simulink model "Final_Model_2025A"  (R2025a)
settings: Solver=VariableStepAuto  StartTime=0.0  StopTime=30  RelTol=1e-3
undefined symbols (not defined in the file): dspblkCoreblockFVToolHelper, gcbh
libraries: dsparch4 x6, dspvision x4, dspsnks4 x1
settings Model: Creator=harry  LastModifiedBy=hr563

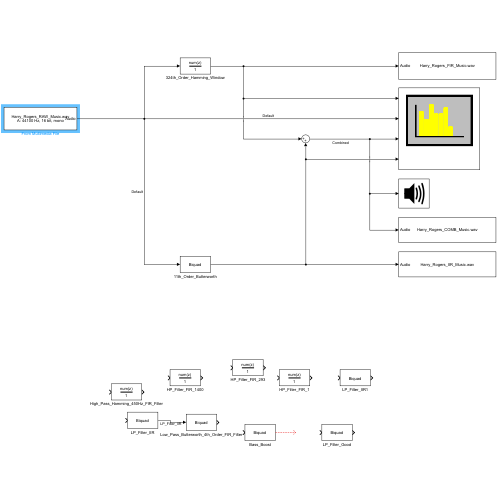
[thumbnail: Simulink's stored preview of the top-level diagram]
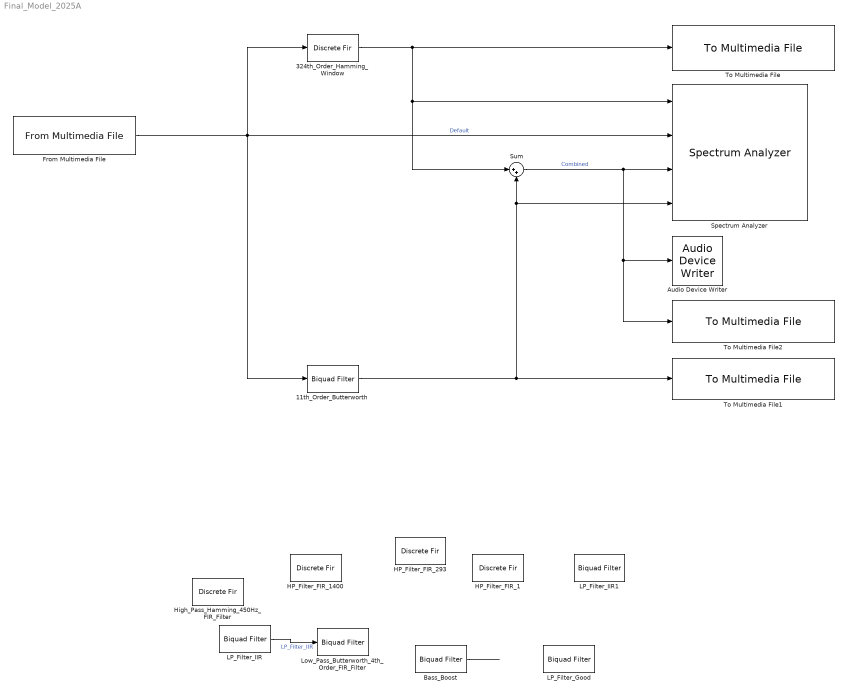
== system Final_Model_2025A ==
  11th_Order_Butterworth : dsparch4/Biquad Filter  Tag=BlockMethodSubSystem  FilterSource=Dialog parameters  CoeffSource=Specify via dialog  FilterObject=BQF  IIRFiltStruct=Direct form II  BiQuadCoeffs=[1 2 1 1 -1.86718651288637583 0.930317821620682883;1 2 1 1 -1.75017085842052844 0.809345759287786626;1 2 1 1 -1.65901358853543979 0.715106377514692082;1 2 1 1 -1.59437049097514039 0.648277636837619742;1 2 1 1 -1.55591215178388231 0.60851898550928496;1 1 0 1 -0.771580047210876474 0]  ScaleValues=[0.0157828271835766983;0.0147937252168145895;0.0140231972448130234;0.0134767864656198163;0.0131517084313506494;0.114209976394561735;1]  IC=0  ICnum=0  ICden=0  a0Flag=Warning  optimizeScaleValues=on  ScaleValueMode=Specify via input port (g)  InputProcessing=Columns as channels (frame based)  roundingMode=Floor  overflowMode=off  scaleValueFracLength=14  denProdOutputFracLength=30  denAccumFracLength=30  secondMemoryFracLength=15
  324th_Order_Hamming_Window : DiscreteFir  Tag=BlockMethodSubSystem  Coefficients=[0.000101883144796532701 6.86919896372373761e-05 3.0551827126106626e-05 -1.03598348954163603e-05 -5.16579270239632391e-05 -9.08628616463472204e-05 -0.000125523401849254363 -0.000153345544928162425 -0.000172322705682308142 -0.0001808615327952031 -0.000177896814554488319 -0.000162988272937909177 -0.000136391758987141042 -9.90975869556805417e-05 -5.28295892007051579e-05 3.67373583371040851e-19 5.63825150002342541e-05 0.000112851545613355976 0.000165664909834257676 0.000211022928791822369 0.000245312472036879933 0.000265363001797536201 0.000268698231497241239 0.000253765330008578279 0.000220123109025119166 0.000168571515594089758 0.000101207108725427596 2.13930078590154471e-05 -6.63630819330360814e-05 -0.000156623005104577644 -0.000243317869524272844 -0.000320119750054912008 -0.000380865129789689934 -0.000420004064119163347 -0.000433044725249857616 -0.000416960561512023258 -0.000370527146366229139 -0.000294558108627706922 -0.00019201436393307482 -6.79680504334934652e-05 7.05882443586693624e-05 0.000215085730591075002 0.000355864481977990078 0.000482775278779599786 0.000585863696247650189 0.000656093174251949737 0.000686057617941617914 0.000670631094018952763 0.000607502860797922524 0.000497550517162741808 0.000345012413622010296 0.000157432285192392427 -5.46362948927894444e-05 -0.000278161469031175032 -0.000498379071641175272 -0.000699714415808812555 -0.000866825914804108871 -0.00098570410124290621 -0.00104475114779683078 -0.0010357624136966496 -0.000954733413222053073 -0.000802423133919360218 -0.000584617630106775408 -0.000312055677203152706 -3.65606249683564421e-17 0.000332538151684784098 0.000663888110730826049 0.000971065241568101474 0.00123129363830265254 0.00142360956883102498 0.00153043758852049573 0.00153902667756687303 0.00144263691875525283 0.00124137834252432836 0.000942622283484140732 0.000560931015285178478 0.000117482131024904072 -0.000361001765768432072 -0.000843772220868447783 -0.00129794307480813687 -0.0016906374133820437 -0.00199125886818211266 -0.00217373660619727196 -0.00221858677488572832 -0.00211463719958366768 -0.00186027704044082454 -0.00146411843666072942 -0.00094499167688704398 -0.000331237214998534777 0.000340695622130973491 0.00102828509125300438 0.00168550368985615059 0.00226576801035194113 0.00272509066434238655 0.0030252296844812134 0.00313662014587347141 0.00304087624971733066 0.00273267024058921172 0.00222082676923184442 0.0015285161619500217 0.000692485083967047787 -0.000238674949218946607 -0.00120715570869207411 -0.00214932764463113832 -0.00299971477484106555 -0.00369531265232305546 -0.00417997777328447256 -0.00440859799464370788 -0.00435075319633216034 -0.00399359443685079994 -0.00334370785079183197 -0.00242778488815178616 -0.0012919903404852379 9.92606710287512014e-17 0.00137023404897434337 0.0027308459883259948 0.00398932091309959873 0.00505436537057680092 0.00584203302811834874 0.00628172024669043216 0.00632163509487150988 0.00593335705089946108 0.00511514350829275332 0.00389370181746993838 0.00232422898026746075 0.000488620844677755198 -0.00150813690696118105 -0.00354326904389297512 -0.00548296361206709534 -0.0071902367066978487 -0.00853348343040164631 -0.00939522672770957447 -0.00968054059413358745 -0.00932461951342663208 -0.0082989932880848296 -0.0066159451763069272 -0.00433077896314346209 -0.00154169294984985664 0.00161285011947875641 0.00495922573952324586 0.00829604582443028982 0.0114035350094972912 0.0140544413260888078 0.016025932931825377 0.0171118565994586753 0.0171346915278984546 0.0159565270886542591 0.0134884265742894315 0.00969760983343864909 0.00461199258818189954 -0.00167824611344687927 -0.00902224159297380576 -0.0172131713291425285 -0.0259959658054706444 -0.0350776695661746893 -0.0441399695405789508 -0.0528532821217139182 -0.0608916968874572279 -0.0679480189210882463 -0.0737481369847406143 -0.0780639725324154959 -0.0807243334855240052 0.918259911176981802 -0.0807243334855240052 -0.0780639725324154959 -0.0737481369847406143 -0.0679480189210882463 -0.0608916968874572279 ...(+3741 chars)]  InputProcessing=Columns as channels (frame based)
  Audio Device Writer : dspsnks4/Audio Device Writer  Driver=DirectSound  Device=Default  InheritSampleRate=on  SampleRate=44100  BitDepth=16-bit integer  BufferSize=4096  NumBuffers=10  DefaultOutputChannelMapping=on  OutputChannelMapping=1:2  OutputNumUnderrunSamples=off  DriverIdx=1  DeviceWarnFlag=''
  Bass_Boost : dsparch4/Biquad Filter  Tag=BlockMethodSubSystem  FilterSource=Dialog parameters  CoeffSource=Specify via dialog  FilterObject=BQF  IIRFiltStruct=Direct form II  BiQuadCoeffs=[1 0 -1 1 -1.97922777247152193 0.979852553935027126;1 0 -1 1 -1.99208152287231277 0.992175167997945806]  ScaleValues=[0.0099035520411623959;0.0099035520411623959;1]  IC=0  ICnum=0  ICden=0  a0Flag=Warning  optimizeScaleValues=on  ScaleValueMode=Specify via input port (g)  InputProcessing=Columns as channels (frame based)  roundingMode=Floor  overflowMode=off  scaleValueFracLength=14  denProdOutputFracLength=30  denAccumFracLength=30  secondMemoryFracLength=15
  From Multimedia File : dspvision/From Multimedia File  inputFilename=C:\Users\hr563\OneDrive - University of Brighton\Year 3\EO626 - Digital Signal Processing\02 - Labs & Coursework\Final Project\Version 2\Harry_Rogers_RAW_Music.wav  readRange=[1 Inf]  loop=on  numPlays=inf  outputStreams=Audio only  videoDataType=single  audioDataType=double  inheritSampleTime=on  userDefinedSampleTime=1/30  noAudioOutput=off  isIntensityVideo=off  fourcc=RGB  colorVideoFormat=Separate color signals  outputEOF=off  dataOrg=Column-major  audioFrameSize=1024  computeAudioFrameSize=off  outSamplingMode=Sample based
      settings: LibrarySourceBlock=audiosources/From Multimedia File
  HP_Filter_FIR_1 : DiscreteFir  Tag=BlockMethodSubSystem  LoadFcn=dspblkCoreblockFVToolHelper(gcbh,'load');  Coefficients=[-0.000172363924315728858 -0.000162411128573225228 -0.000141952632408346325 -0.000111937875448206057 -7.3851199371037808e-05 -2.9665348286780504e-05 1.82276088386097535e-05 6.71088533093024717e-05 0.000114048947032513665 0.000156046191835491031 0.000190184041238055756 0.000213802202744505318 0.000224673747451289524 0.000221178337738877408 0.000202459872990196294 0.000168555718425642166 0.00012048447429225332 6.028015285343048e-05 -9.0372368165297075e-06 -8.35613444034827242e-05 -0.000158671573688910707 -0.00022927451432170617 -0.000290105803670732206 -0.00033607765210802253 -0.000362651848377851607 -0.000366213607692528946 -0.000344418626364605509 -0.000296484582778010057 -0.000223399378251365769 -0.000128021791785200718 -1.50558976478667982e-05 0.000109111662719308189 0.000236713072915811486 0.000359030473486977799 0.000466937148628223774 0.000551518831532300346 0.00060473630847924717 0.000620083808060237435 0.000593193875587250813 0.000522339099862775304 0.000408784497940755179 0.000256951620138050395 7.43662639955295377e-05 -0.000128624463839541327 -0.000339363947310907747 -0.000543607733929659981 -0.000726418970532887506 -0.000873185750649687546 -0.00097069545809302135 -0.00100819198737314882 -0.000978337351840312657 -0.000878000331284546111 -0.000708801768935293699 -0.000477358793517133125 -0.000195188069684670715 0.000121749798270892953 0.000453857713884555042 0.000779028316384048161 0.00107403047870383993 0.00131607467262399532 0.00148445729625005574 0.00156217158522543474 0.00153736757952660334 0.00140454663245319919 0.00116538742266552317 0.000829120060655970186 0.000412391753901741398 -6.1399883169818039e-05 -0.000563293414391254467 -0.00106041986086509075 -0.00151804198472996221 -0.00190185733672405539 -0.00218041976363849256 -0.00232751673198150662 -0.0023243329454521555 -0.00216123540699293031 -0.00183903163276229165 -0.00136958067386139899 -0.000775674619164995385 -9.01542351587077237e-05 0.000645726430807490163 0.00138461858811187648 0.00207596111382843222 0.0026692615626617653 0.00311757334470875091 0.00338094138492120054 0.00342957760910434211 0.00324653243692826689 0.0028296496090265558 0.00219262854278050659 0.00136506930185104698 0.000391437435900149648 -0.000671044248027770178 -0.00175549682802994393 -0.00278932756878535072 -0.00369879642900174674 -0.00441393573992427627 -0.00487351324290121596 -0.00502970856114155936 -0.00485217399934524153 -0.00433117329036738705 -0.0034795361035329553 -0.00233322991392799408 -0.000950430945598244176 0.00059093213758860052 0.00219708976874827787 0.00376362758981319207 0.0051817039743920143 0.00634494566982728332 0.00715661624830996653 0.00753661293967718832 0.00742783471297681595 0.00680148013467851177 0.00566087777367077494 0.00404352314560369255 0.00202109101148037224 -0.000302694738201085491 -0.00279632574162053766 -0.00530677000518562855 -0.00766746317937382679 -0.00970764829638974015 -0.0112625845722653661 -0.012184074032272273 -0.0123507139156610306 -0.0116772768537853379 -0.0101226515937356768 -0.00769584445638855572 -0.00445964373969970612 -0.00053168220654616744 0.00391720821819646972 0.00866727552988320188 0.0134564898180329438 0.0179890652298531316 0.0219451435763498778 0.0249906435928888039 0.0267859088499742271 0.0269912108286908779 0.0252661306287800883 0.0212577699554858598 0.0145681863422995467 0.00468052310781379068 -0.00920564171979430454 -0.0285662975876889227 -0.0566203819789594456 -0.101953907686601439 -0.196616698385724042 -0.631266180659922238 0.631266180659922238 0.196616698385724042 0.101953907686601439 0.0566203819789594456 0.0285662975876889227 0.00920564171979430454 -0.00468052310781379068 -0.0145681863422995467 -0.0212577699554858598 -0.0252661306287800883 -0.0269912108286908779 -0.0267859088499742271 -0.0249906435928888039 -0.0219451435763498778 -0.0179890652298531316 -0.0134564898180329438 -0.00866727552988320188 -0.00391720821819646972 0.00053168220654616744 0.00445964373969970612 0.00769584445638855572 0.0101226515937356768 ...(+2982 chars)]  InputProcessing=Columns as channels (frame based)
      settings: CopyFcn=dspblkCoreblockFVToolHelper(gcbh,'copy');  DeleteFcn=dspblkCoreblockFVToolHelper(gcbh,'close');  ModelCloseFcn=dspblkCoreblockFVToolHelper(gcbh,'close');  PreSaveFcn=dspblkCoreblockFVToolHelper(gcbh,'presave');  PostSaveFcn=dspblkCoreblockFVToolHelper(gcbh,'postsave');  CloseFcn=dspblkCoreblockFVToolHelper(gcbh,'close');
  HP_Filter_FIR_1400 : DiscreteFir  Tag=BlockMethodSubSystem  Coefficients=[-3.41011682905011137e-05 -3.10559172244132767e-05 -2.59704425703152653e-05 -1.91699897519594766e-05 -1.10922885580064924e-05 -2.25957592028960039e-06 6.75493320791177441e-06 1.5363989756872894e-05 2.30043051885164215e-05 2.91731560537851625e-05 3.34612364628995916e-05 3.55796265981361698e-05 3.53791128579665512e-05 3.28605772797087772e-05 2.817574042505612e-05 2.16181572859737575e-05 1.36049910339950962e-05 4.65068479285764637e-06 -4.6658210837113406e-06 -1.37382535674786507e-05 -2.19721854293832492e-05 -2.88237141255762545e-05 -3.38351420219722165e-05 -3.66653335945134315e-05 -3.71127502897256254e-05 -3.51296195208254772e-05 -3.08262527275190195e-05 -2.44651536838152741e-05 -1.64452128142218818e-05 -7.27692453362485335e-06 2.44984861227346711e-06 1.21035470412975323e-05 2.10516334209167097e-05 2.87017539985367584e-05 3.45406822275087029e-05 3.81685019521315502e-05 3.93257692886763203e-05 3.79118227132474732e-05 3.39929636933614958e-05 2.77998712973231524e-05 1.97143033587088446e-05 1.02458301928054272e-05 -1.43291443473674532e-18 -1.03600945567594416e-05 -2.01564292519422879e-05 -2.87401223854129503e-05 -3.55341248592242601e-05 -4.00717364834981459e-05 -4.20283952608714961e-05 -4.12445910286335254e-05 -3.77383036428625458e-05 -3.17060253166553859e-05 -2.35121556387111352e-05 -1.36673100192635751e-05 -2.79680951490947161e-06 8.39872521177538563e-06 1.91882140173775877e-05 2.88575429812699572e-05 3.67565199570511276e-05 4.23422925095269241e-05 4.5216348115168936e-05 4.51525936634749101e-05 4.21145565924994767e-05 3.62604305214517085e-05 2.79354618385117793e-05 1.76519915136439117e-05 6.05827596191914808e-06 -6.10204067022114899e-06 -1.80372925035369491e-05 -2.89590018398164513e-05 -3.81336422904404674e-05 -4.49315780750668805e-05 -4.88699350290324068e-05 -4.96465052091935567e-05 -4.71623279491193041e-05 -4.15312936419230796e-05 -3.30759391668579956e-05 -2.23094939846204235e-05 -9.90513650925184875e-06 3.345727209407499e-06 1.65836026605182578e-05 2.89363114943004043e-05 3.95761131366971562e-05 4.77748246071605157e-05 5.2953290051345063e-05 5.47218618906218475e-05 5.29090897148440042e-05 4.75765399293508288e-05 3.90185443937111727e-05 2.77466450637399063e-05 1.44595020988057325e-05 -1.18271311595691961e-18 -1.4697843873563345e-05 -2.86688503206844876e-05 -4.09797025741088575e-05 -5.07909318547471202e-05 -5.74137706463406609e-05 -6.03580474054663733e-05 -5.93678196977923654e-05 -5.44421921531140565e-05 -4.58396959021705236e-05 -3.40656593559356003e-05 -1.98431092620320828e-05 -4.0688340026943614e-06 1.22427540683630008e-05 2.80244714637696102e-05 4.22258112556728377e-05 5.38824907874365126e-05 6.21815193377174091e-05 6.65174204924286102e-05 6.65357500618489879e-05 6.21608195978629133e-05 5.36055219630269039e-05 4.13622978888251875e-05 2.61755085599021872e-05 8.99670967999697371e-06 -9.07452379900674041e-06 -2.68605734952090588e-05 -4.31821283474038999e-05 -5.69359858632199542e-05 -6.71691965022533729e-05 -7.31445945383622976e-05 -7.43932391404152651e-05 -7.07500737262434655e-05 -6.23701535911282064e-05 -4.97240272600675692e-05 -3.3572207898318735e-05 -1.49200503392781792e-05 5.04433369426768165e-06 2.50253228685259366e-05 4.37034600126417734e-05 5.98221757188546798e-05 7.22718881018664206e-05 8.01658775142756556e-05 8.29027787878004025e-05 8.02113259973277195e-05 7.21740797205544483e-05 5.92281973553958766e-05 4.21427895438527663e-05 2.19739448675932221e-05 -2.99731528384923268e-18 -2.23590162023749559e-05 -4.36327205209957573e-05 -6.23966489100494638e-05 -7.73671897462060315e-05 -8.74888783155105995e-05 -9.20081476517277489e-05 -9.05284218871913311e-05 -8.30425815327852059e-05 -6.99402562086595512e-05 -5.19890199878336265e-05 -3.02902739761851766e-05 -6.21228852709459262e-06 1.86955684798287861e-05 4.28020757771411278e-05 6.45005488484745853e-05 8.2315465957998396e-05 9.50022831821261413e-05 0.000101633718625495422 0.000101666563444777433 9.49842615824907457e-05 8.19120199887399361e-05 6.32029718649274248e-05 ...(+31187 chars)]  InputProcessing=Columns as channels (frame based)
  HP_Filter_FIR_293 : DiscreteFir  Tag=BlockMethodSubSystem  LoadFcn=dspblkCoreblockFVToolHelper(gcbh,'load');  Coefficients=[-0.000172363924315728858 -0.000162411128573225228 -0.000141952632408346325 -0.000111937875448206057 -7.3851199371037808e-05 -2.9665348286780504e-05 1.82276088386097535e-05 6.71088533093024717e-05 0.000114048947032513665 0.000156046191835491031 0.000190184041238055756 0.000213802202744505318 0.000224673747451289524 0.000221178337738877408 0.000202459872990196294 0.000168555718425642166 0.00012048447429225332 6.028015285343048e-05 -9.0372368165297075e-06 -8.35613444034827242e-05 -0.000158671573688910707 -0.00022927451432170617 -0.000290105803670732206 -0.00033607765210802253 -0.000362651848377851607 -0.000366213607692528946 -0.000344418626364605509 -0.000296484582778010057 -0.000223399378251365769 -0.000128021791785200718 -1.50558976478667982e-05 0.000109111662719308189 0.000236713072915811486 0.000359030473486977799 0.000466937148628223774 0.000551518831532300346 0.00060473630847924717 0.000620083808060237435 0.000593193875587250813 0.000522339099862775304 0.000408784497940755179 0.000256951620138050395 7.43662639955295377e-05 -0.000128624463839541327 -0.000339363947310907747 -0.000543607733929659981 -0.000726418970532887506 -0.000873185750649687546 -0.00097069545809302135 -0.00100819198737314882 -0.000978337351840312657 -0.000878000331284546111 -0.000708801768935293699 -0.000477358793517133125 -0.000195188069684670715 0.000121749798270892953 0.000453857713884555042 0.000779028316384048161 0.00107403047870383993 0.00131607467262399532 0.00148445729625005574 0.00156217158522543474 0.00153736757952660334 0.00140454663245319919 0.00116538742266552317 0.000829120060655970186 0.000412391753901741398 -6.1399883169818039e-05 -0.000563293414391254467 -0.00106041986086509075 -0.00151804198472996221 -0.00190185733672405539 -0.00218041976363849256 -0.00232751673198150662 -0.0023243329454521555 -0.00216123540699293031 -0.00183903163276229165 -0.00136958067386139899 -0.000775674619164995385 -9.01542351587077237e-05 0.000645726430807490163 0.00138461858811187648 0.00207596111382843222 0.0026692615626617653 0.00311757334470875091 0.00338094138492120054 0.00342957760910434211 0.00324653243692826689 0.0028296496090265558 0.00219262854278050659 0.00136506930185104698 0.000391437435900149648 -0.000671044248027770178 -0.00175549682802994393 -0.00278932756878535072 -0.00369879642900174674 -0.00441393573992427627 -0.00487351324290121596 -0.00502970856114155936 -0.00485217399934524153 -0.00433117329036738705 -0.0034795361035329553 -0.00233322991392799408 -0.000950430945598244176 0.00059093213758860052 0.00219708976874827787 0.00376362758981319207 0.0051817039743920143 0.00634494566982728332 0.00715661624830996653 0.00753661293967718832 0.00742783471297681595 0.00680148013467851177 0.00566087777367077494 0.00404352314560369255 0.00202109101148037224 -0.000302694738201085491 -0.00279632574162053766 -0.00530677000518562855 -0.00766746317937382679 -0.00970764829638974015 -0.0112625845722653661 -0.012184074032272273 -0.0123507139156610306 -0.0116772768537853379 -0.0101226515937356768 -0.00769584445638855572 -0.00445964373969970612 -0.00053168220654616744 0.00391720821819646972 0.00866727552988320188 0.0134564898180329438 0.0179890652298531316 0.0219451435763498778 0.0249906435928888039 0.0267859088499742271 0.0269912108286908779 0.0252661306287800883 0.0212577699554858598 0.0145681863422995467 0.00468052310781379068 -0.00920564171979430454 -0.0285662975876889227 -0.0566203819789594456 -0.101953907686601439 -0.196616698385724042 -0.631266180659922238 0.631266180659922238 0.196616698385724042 0.101953907686601439 0.0566203819789594456 0.0285662975876889227 0.00920564171979430454 -0.00468052310781379068 -0.0145681863422995467 -0.0212577699554858598 -0.0252661306287800883 -0.0269912108286908779 -0.0267859088499742271 -0.0249906435928888039 -0.0219451435763498778 -0.0179890652298531316 -0.0134564898180329438 -0.00866727552988320188 -0.00391720821819646972 0.00053168220654616744 0.00445964373969970612 0.00769584445638855572 0.0101226515937356768 ...(+2982 chars)]  InputProcessing=Columns as channels (frame based)
      settings: CopyFcn=dspblkCoreblockFVToolHelper(gcbh,'copy');  DeleteFcn=dspblkCoreblockFVToolHelper(gcbh,'close');  ModelCloseFcn=dspblkCoreblockFVToolHelper(gcbh,'close');  PreSaveFcn=dspblkCoreblockFVToolHelper(gcbh,'presave');  PostSaveFcn=dspblkCoreblockFVToolHelper(gcbh,'postsave');  CloseFcn=dspblkCoreblockFVToolHelper(gcbh,'close');
  High_Pass_Hamming_450Hz_FIR_Filter : DiscreteFir  Tag=BlockMethodSubSystem  Coefficients=[0.000101883144796532701 6.86919896372373761e-05 3.0551827126106626e-05 -1.03598348954163603e-05 -5.16579270239632391e-05 -9.08628616463472204e-05 -0.000125523401849254363 -0.000153345544928162425 -0.000172322705682308142 -0.0001808615327952031 -0.000177896814554488319 -0.000162988272937909177 -0.000136391758987141042 -9.90975869556805417e-05 -5.28295892007051579e-05 3.67373583371040851e-19 5.63825150002342541e-05 0.000112851545613355976 0.000165664909834257676 0.000211022928791822369 0.000245312472036879933 0.000265363001797536201 0.000268698231497241239 0.000253765330008578279 0.000220123109025119166 0.000168571515594089758 0.000101207108725427596 2.13930078590154471e-05 -6.63630819330360814e-05 -0.000156623005104577644 -0.000243317869524272844 -0.000320119750054912008 -0.000380865129789689934 -0.000420004064119163347 -0.000433044725249857616 -0.000416960561512023258 -0.000370527146366229139 -0.000294558108627706922 -0.00019201436393307482 -6.79680504334934652e-05 7.05882443586693624e-05 0.000215085730591075002 0.000355864481977990078 0.000482775278779599786 0.000585863696247650189 0.000656093174251949737 0.000686057617941617914 0.000670631094018952763 0.000607502860797922524 0.000497550517162741808 0.000345012413622010296 0.000157432285192392427 -5.46362948927894444e-05 -0.000278161469031175032 -0.000498379071641175272 -0.000699714415808812555 -0.000866825914804108871 -0.00098570410124290621 -0.00104475114779683078 -0.0010357624136966496 -0.000954733413222053073 -0.000802423133919360218 -0.000584617630106775408 -0.000312055677203152706 -3.65606249683564421e-17 0.000332538151684784098 0.000663888110730826049 0.000971065241568101474 0.00123129363830265254 0.00142360956883102498 0.00153043758852049573 0.00153902667756687303 0.00144263691875525283 0.00124137834252432836 0.000942622283484140732 0.000560931015285178478 0.000117482131024904072 -0.000361001765768432072 -0.000843772220868447783 -0.00129794307480813687 -0.0016906374133820437 -0.00199125886818211266 -0.00217373660619727196 -0.00221858677488572832 -0.00211463719958366768 -0.00186027704044082454 -0.00146411843666072942 -0.00094499167688704398 -0.000331237214998534777 0.000340695622130973491 0.00102828509125300438 0.00168550368985615059 0.00226576801035194113 0.00272509066434238655 0.0030252296844812134 0.00313662014587347141 0.00304087624971733066 0.00273267024058921172 0.00222082676923184442 0.0015285161619500217 0.000692485083967047787 -0.000238674949218946607 -0.00120715570869207411 -0.00214932764463113832 -0.00299971477484106555 -0.00369531265232305546 -0.00417997777328447256 -0.00440859799464370788 -0.00435075319633216034 -0.00399359443685079994 -0.00334370785079183197 -0.00242778488815178616 -0.0012919903404852379 9.92606710287512014e-17 0.00137023404897434337 0.0027308459883259948 0.00398932091309959873 0.00505436537057680092 0.00584203302811834874 0.00628172024669043216 0.00632163509487150988 0.00593335705089946108 0.00511514350829275332 0.00389370181746993838 0.00232422898026746075 0.000488620844677755198 -0.00150813690696118105 -0.00354326904389297512 -0.00548296361206709534 -0.0071902367066978487 -0.00853348343040164631 -0.00939522672770957447 -0.00968054059413358745 -0.00932461951342663208 -0.0082989932880848296 -0.0066159451763069272 -0.00433077896314346209 -0.00154169294984985664 0.00161285011947875641 0.00495922573952324586 0.00829604582443028982 0.0114035350094972912 0.0140544413260888078 0.016025932931825377 0.0171118565994586753 0.0171346915278984546 0.0159565270886542591 0.0134884265742894315 0.00969760983343864909 0.00461199258818189954 -0.00167824611344687927 -0.00902224159297380576 -0.0172131713291425285 -0.0259959658054706444 -0.0350776695661746893 -0.0441399695405789508 -0.0528532821217139182 -0.0608916968874572279 -0.0679480189210882463 -0.0737481369847406143 -0.0780639725324154959 -0.0807243334855240052 0.918259911176981802 -0.0807243334855240052 -0.0780639725324154959 -0.0737481369847406143 -0.0679480189210882463 -0.0608916968874572279 ...(+3741 chars)]  InputProcessing=Columns as channels (frame based)
  LP_Filter_Good : dsparch4/Biquad Filter  Tag=BlockMethodSubSystem  FilterSource=Dialog parameters  CoeffSource=Specify via dialog  FilterObject=BQF  IIRFiltStruct=Direct form II  BiQuadCoeffs=[1 2 1 1 -1.76341598268706057 0.823038713497136087;1 2 1 1 -1.56729903101675361 0.620290865695949267]  ScaleValues=[0.0149056827025188555;0.0132479586697988976;1]  IC=0  ICnum=0  ICden=0  a0Flag=Warning  optimizeScaleValues=on  ScaleValueMode=Specify via input port (g)  InputProcessing=Columns as channels (frame based)  roundingMode=Floor  overflowMode=off  scaleValueFracLength=14  denProdOutputFracLength=30  denAccumFracLength=30  secondMemoryFracLength=15
  LP_Filter_IIR : dsparch4/Biquad Filter  Tag=BlockMethodSubSystem  FilterSource=Dialog parameters  CoeffSource=Specify via dialog  FilterObject=BQF  IIRFiltStruct=Direct form II  BiQuadCoeffs=[1 2 1 1 -1.83393339064791361 0.886044963112266548;1 2 1 1 -1.6692031429311931 0.716633873504157637;1 2 1 1 -1.5869067908315011 0.631999054621612988]  ScaleValues=[0.0130278931160882541;0.0118576826432411561;0.011273065947527923;1]  IC=0  ICnum=0  ICden=0  a0Flag=Warning  optimizeScaleValues=on  ScaleValueMode=Specify via input port (g)  InputProcessing=Columns as channels (frame based)  roundingMode=Floor  overflowMode=off  scaleValueFracLength=14  denProdOutputFracLength=30  denAccumFracLength=30  secondMemoryFracLength=15
  LP_Filter_IIR1 : dsparch4/Biquad Filter  Tag=BlockMethodSubSystem  FilterSource=Dialog parameters  CoeffSource=Specify via dialog  FilterObject=BQF  IIRFiltStruct=Direct form II  BiQuadCoeffs=[1 2 1 1 -1.83393339064791361 0.886044963112266548;1 2 1 1 -1.6692031429311931 0.716633873504157637;1 2 1 1 -1.5869067908315011 0.631999054621612988]  ScaleValues=[0.0130278931160882541;0.0118576826432411561;0.011273065947527923;1]  IC=0  ICnum=0  ICden=0  a0Flag=Warning  optimizeScaleValues=on  ScaleValueMode=Specify via input port (g)  InputProcessing=Columns as channels (frame based)  roundingMode=Floor  overflowMode=off  scaleValueFracLength=14  denProdOutputFracLength=30  denAccumFracLength=30  secondMemoryFracLength=15
  Low_Pass_Butterworth_4th_Order_FIR_Filter : dsparch4/Biquad Filter  Tag=BlockMethodSubSystem  FilterSource=Dialog parameters  CoeffSource=Specify via dialog  FilterObject=BQF  IIRFiltStruct=Direct form II  BiQuadCoeffs=[1 2 1 1 -1.76341598268706057 0.823038713497136087;1 2 1 1 -1.56729903101675361 0.620290865695949267]  ScaleValues=[0.0149056827025188555;0.0132479586697988976;1]  IC=0  ICnum=0  ICden=0  a0Flag=Warning  optimizeScaleValues=on  ScaleValueMode=Specify via input port (g)  InputProcessing=Columns as channels (frame based)  roundingMode=Floor  overflowMode=off  scaleValueFracLength=14  denProdOutputFracLength=30  denAccumFracLength=30  secondMemoryFracLength=15
  Spectrum Analyzer : SpectrumAnalyzer  NumInputPorts=4  WindowPosition=[130.000000,32.000000,1675.000000,849.000000,]  ScopeFrameLocation=window  SampleRate=44.1e3  FrequencyScale=Log  WindowInvariantSamplesPerUpdate=on  FrequencySpan=Start and stop frequencies  StartFrequency=20  StopFrequency=22050  MaximizeAxes=Off  YLimits=[-277.2722 31.5803]  ShowLegend=on  ExpandToolstrip=on  SelectedToolstripTab=spectrumAnalyzerToolstrip.channelMeasurementsTab  MeasurementChannel=0
  Sum : Sum  Inputs=|++
  To Multimedia File : dspvision/To Multimedia File  outputFilename=Harry_Rogers_FIR_Music.wav  streamSelection=Audio only  videoCompressor=None (uncompressed)  audioCompressor=None (uncompressed)  imagePorts=One multidimensional signal  fileType=WAV  audioDatatype=16-bit integer  fourcc=RGB  audioBitRate=128  audioQuality=75  videoQuality=75  mj2000CompFactor=10
      settings: LibrarySourceBlock=audiosinks/To Multimedia File
  To Multimedia File1 : dspvision/To Multimedia File  outputFilename=Harry_Rogers_IIR_Music.wav  streamSelection=Audio only  videoCompressor=None (uncompressed)  audioCompressor=None (uncompressed)  imagePorts=One multidimensional signal  fileType=WAV  audioDatatype=16-bit integer  fourcc=RGB  audioBitRate=128  audioQuality=75  videoQuality=75  mj2000CompFactor=10
      settings: LibrarySourceBlock=audiosinks/To Multimedia File
  To Multimedia File2 : dspvision/To Multimedia File  outputFilename=Harry_Rogers_COMB_Music.wav  streamSelection=Audio only  videoCompressor=None (uncompressed)  audioCompressor=None (uncompressed)  imagePorts=One multidimensional signal  fileType=WAV  audioDatatype=16-bit integer  fourcc=RGB  audioBitRate=128  audioQuality=75  videoQuality=75  mj2000CompFactor=10
      settings: LibrarySourceBlock=audiosinks/To Multimedia File
  wires:
  From Multimedia File/1 -> 11th_Order_Butterworth/1, 324th_Order_Hamming_Window/1, Spectrum Analyzer/2  "Default"
  11th_Order_Butterworth/1 -> To Multimedia File1/1, Spectrum Analyzer/4, Sum/2
  Sum/1 -> To Multimedia File2/1, Audio Device Writer/1, Spectrum Analyzer/3  "Combined"
  324th_Order_Hamming_Window/1 -> Sum/1, Spectrum Analyzer/1, To Multimedia File/1
  Bass_Boost/1 -> ?
  LP_Filter_IIR/1 -> Low_Pass_Butterworth_4th_Order_FIR_Filter/1  "LP_Filter_IIR"
